simulink model "malt_mot_test"  (R2023a)
settings: Solver=FixedStepAuto  StartTime=0.0  StopTime=50  FixedStep=framePeriod_s  RelTol=1e-3
undefined symbols (not defined in the file or in its folder): Aircraft, framePeriod_s
settings Model: Creator=brian  LastModifiedBy=tuan
settings SolverCC: AlgebraicLoopSolver=TrustRegion
settings OptimizationCC: DefaultParameterBehavior=Inlined  GainParamInheritBuiltInType=on  UseFloatMulNetSlope=on  DefaultUnderspecifiedDataType=single  EnhancedBackFolding=on  BooleansAsBitfields=on  PassReuseOutputArgsAs=Individual arguments  StateBitsets=on  DataBitsets=on  ActiveStateOutputEnumStorageType=uint16  ZeroExternalMemoryAtStartup=off  ZeroInternalMemoryAtStartup=off  EfficientFloat2IntCast=on  LifeSpan=inf  DifferentSizesBufferReuse=on  OptimizationPriority=RAM  OptimizationCustomize=off  EfficientTunableParamExpr=on
settings DebuggingCC: ParameterPrecisionLossMsg=none  ParameterTunabilityLossMsg=error  UnconnectedInputMsg=warning  UnconnectedOutputMsg=warning  UnconnectedLineMsg=warning  BusObjectLabelMismatch=error  RootOutportRequireBusObject=error  NonBusSignalsTreatedAsBus=error  SFInvalidInputDataAccessInChartInitDiag=error  SFTransitionOutsideNaturalParentDiag=error  SFUnreachableExecutionPathDiag=error  SFUndirectedBroadcastEventsDiag=error
settings HardwareCC: ProdBitPerPointer=32  ProdBitPerSizeT=32  ProdBitPerPtrDiffT=32  ProdLargestAtomicInteger=Long  ProdLargestAtomicFloat=Double  ProdWordSize=32  ProdHWDeviceType=NXP->Cortex-M4  TargetLargestAtomicInteger=Long  TargetLargestAtomicFloat=Double  TargetLongLongMode=on  TargetIntDivRoundTo=Zero  TargetEndianess=LittleEndian  TargetHWDeviceType=NXP->Cortex-M4  ProdEqTarget=off
settings ModelReferenceCC: EnableRefExpFcnMdlSchedulingChecks=on  ModelReferenceNumInstancesAllowed=Single
settings SFSimCC: SimParseCustomCode=off  SimGenImportedTypeDefs=on  MATLABDynamicMemAlloc=off  SimTargetLang=C++
settings SFSimCC: SimUserIncludeDirs=|
  | ../../flight_code/include
  | ../../../ua_spaaro_extra/imu/include
  | ../../../ua_spaaro_extra/gnss/include
  | ../../../ua_spaaro_extra/pres/include
  | ../../../ua_spaaro_extra/sbus/include
  | ../../../ua_spaaro_extra/global_defs/include
settings SFSimCC: SimUserDefines=|
  | SIL
  | __FMU_R_MINI_V1__
settings RTWCC: Description=Embedded Coder  SystemTargetFile=ert.tlc  GenCodeOnly=on  TemplateMakefile=ert_default_tmf  GenerateReport=on  RTWVerbose=off  RTWUseSimCustomCode=on  Toolchain=GNU gcc/g++ | gmake (64-bit Linux)  BuildConfiguration=Specify  IncludeHyperlinkInReport=on  LaunchReport=on  TargetLang=C++  GenerateTraceInfo=on  GenerateTraceReport=on  GenerateTraceReportSl=on  GenerateTraceReportSf=on  GenerateTraceReportEml=on  GenerateCodeReplacementReport=on  DLArmComputeVersion=19.05
settings RTWCC: CustomInclude=|
  | ../../flight_code/include
  | ../../../ua_spaaro_extra/imu/include
  | ../../../ua_spaaro_extra/gnss/include
  | ../../../ua_spaaro_extra/pres/include
  | ../../../ua_spaaro_extra/sbus/include
  | ../../../ua_spaaro_extra/global_defs/include
settings RTWCC: CustomDefine=|
  | SIL
  | __FMU_R_MINI_V1__
settings CodeAppCC: ForceParamTrailComments=on  IgnoreCustomStorageClasses=off  OperatorAnnotations=on  SimulinkDataObjDesc=on  SFDataObjDesc=on  MATLABFcnDesc=on  CustomSymbolStrGlobalVar=rt$N$M  CustomSymbolStrType=$N$M  CustomSymbolStrFcn=$N$M$F  CustomSymbolStrMacro=$N$M  InsertBlockDesc=on  StateflowObjectComments=on  MATLABSourceComments=on  EnableCustomComments=on  InternalIdentifier=Classic  InlinedPrmAccess=Macros  ReqsInCode=on
settings ERTTargetCC: TargetLangStandard=C++03 (ISO)  GenerateFullHeader=off  IncludeMdlTerminateFcn=off  CombineSignalStateStructs=on  SuppressErrorStatus=on  SupportAbsoluteTime=off  CodeInterfacePackaging=C++ class  SupportNonFinite=off  SupportComplex=off  ParenthesesLevel=Standards  CastingMode=Standards  ERTHeaderFileRootName=autocode$E  ERTSourceFileRootName=autocode$E  InlinedParameterPlacement=NonHierarchical  RootIOFormat=Structure reference  ERTCustomFileTemplate=example_file_process.tlc  ERTFilePackagingFormat=Compact  PreserveExpressionOrder=on  PreserveIfCondition=on  ConvertIfToSwitch=off  EnableSignedLeftShifts=off  EnableSignedRightShifts=off  IndentSize=4

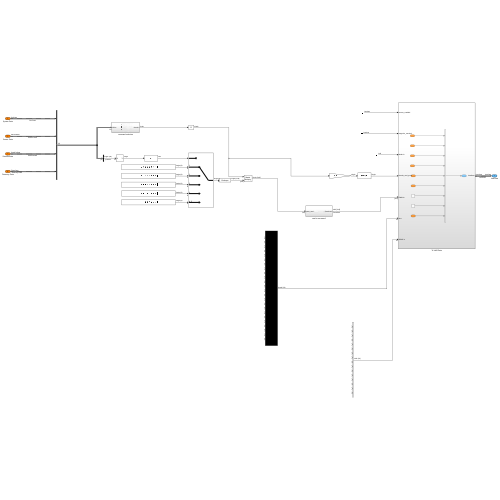
[thumbnail: Simulink's stored preview of the top-level diagram]
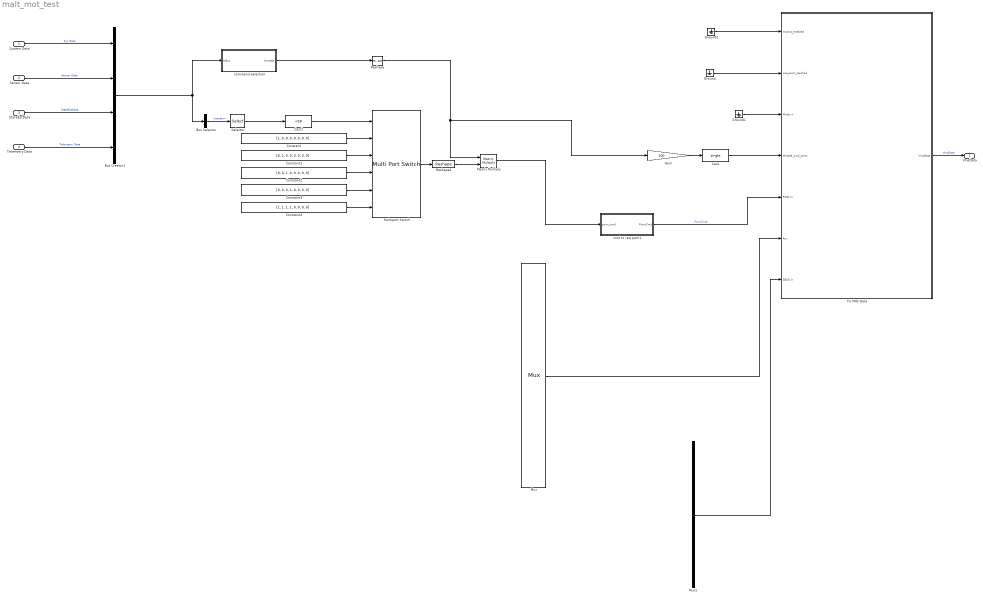
== system malt_mot_test ==
  System Data : Inport  OutDataTypeStr=Bus: SysData  SampleTime=framePeriod_s  BusOutputAsStruct=on
  Sensor Data : Inport  Port=2  OutDataTypeStr=Bus: SensorData  SampleTime=framePeriod_s  BusOutputAsStruct=on
  StateEstData : Inport  Port=3  OutDataTypeStr=Bus: StateEstData  SampleTime=framePeriod_s  BusOutputAsStruct=on
  Telemetry Data : Inport  Port=4  OutDataTypeStr=Bus: TelemData  SampleTime=framePeriod_s  BusOutputAsStruct=on
  Bus Creator1 : BusCreator  Inputs=4
  Bus Selector : BusSelector  OutputSignals=Telemetry Data.param
  Cast : DataTypeConversion  OutDataTypeStr=single  SaturateOnIntegerOverflow=off  RndMeth=Floor
  Cast1 : DataTypeConversion  OutDataTypeStr=int8  SaturateOnIntegerOverflow=off  RndMeth=Floor
  Constant : Constant  Value=[1, 0, 0, 0, 0, 0, 0, 0]  OutDataTypeStr=single  SampleTime=framePeriod_s
  Constant1 : Constant  Value=[0, 1, 0, 0, 0, 0, 0, 0]  OutDataTypeStr=single  SampleTime=framePeriod_s
  Constant2 : Constant  Value=[0, 0, 1, 0, 0, 0, 0, 0]  OutDataTypeStr=single  SampleTime=framePeriod_s
  Constant3 : Constant  Value=[0, 0, 0, 1, 0, 0, 0, 0]  OutDataTypeStr=single  SampleTime=framePeriod_s
  Constant4 : Constant  Value=[1, 1, 1, 1, 0, 0, 0, 0]  OutDataTypeStr=single  SampleTime=framePeriod_s
  Gain : Gain  Gain=100
  Ground : Ground
  Ground1 : Ground
  Ground2 : Ground
  Matrix Multiply : Product  Multiplication=Matrix(*)
  Multiport Switch : MultiPortSwitch  DataPortOrder=Specify indices  DataPortIndices={1, 2, 3, 4, 0}  SaturateOnIntegerOverflow=off  InputSameDT=off
  Mux : Mux  Inputs=24
  Mux1 : Mux  Inputs=16
  Reshape : Reshape  OutputDimensionality=Customize
  Reshape1 : Reshape  OutputDimensionality=Customize  OutputDimensions=[1,8]
  Selector : Selector  IndexMode=Zero-based  InputPortWidth=24  IndexOptions=Index vector (dialog)  Indices=0  OutputSizes=1
  To VMS Data : Subsystem
  cmd to raw pwm1 : Subsystem
  command selection : Subsystem
  VmsData : Outport  OutDataTypeStr=Bus: VmsData  SampleTime=framePeriod_s  BusOutputAsStruct=on
  wires:
  To VMS Data/1(VmsData) -> VmsData/1  "VmsData"
  Ground1/1 -> To VMS Data/3(Mode in)
  Ground2/1 -> To VMS Data/1(motors_enabled)
  Cast/1 -> To VMS Data/4(throttle_cmd_prcnt)
  Reshape/1 -> Gain/1, Matrix Multiply/1
  Gain/1 -> Cast/1
  command selection/1(throttle) -> Reshape/1
  Bus Creator1/1 -> Bus Selector/1, command selection/1(InBus)
  cmd to raw pwm1/1(PwmCmd) -> To VMS Data/5(PWM In)  "PwmCmd"
  Matrix Multiply/1 -> cmd to raw pwm1/1(pwm_cmd)
  Mux/1 -> To VMS Data/6(Aux)
  System Data/1 -> Bus Creator1/1  "Sys Data"
  Sensor Data/1 -> Bus Creator1/2  "Sensor Data"
  StateEstData/1 -> Bus Creator1/3  "StateEstData"
  Mux1/1 -> To VMS Data/7(SBUS in)
  Telemetry Data/1 -> Bus Creator1/4  "Telemetry Data"
  Ground/1 -> To VMS Data/2(waypoint_reached)
  Bus Selector/1 -> Selector/1  "<param>"
  Selector/1 -> Cast1/1
  Constant/1 -> Multiport Switch/2
  Constant1/1 -> Multiport Switch/3
  Constant4/1 -> Multiport Switch/6
  Constant3/1 -> Multiport Switch/5
  Constant2/1 -> Multiport Switch/4
  Multiport Switch/1 -> Reshape1/1
  Cast1/1 -> Multiport Switch/1
  Reshape1/1 -> Matrix Multiply/2

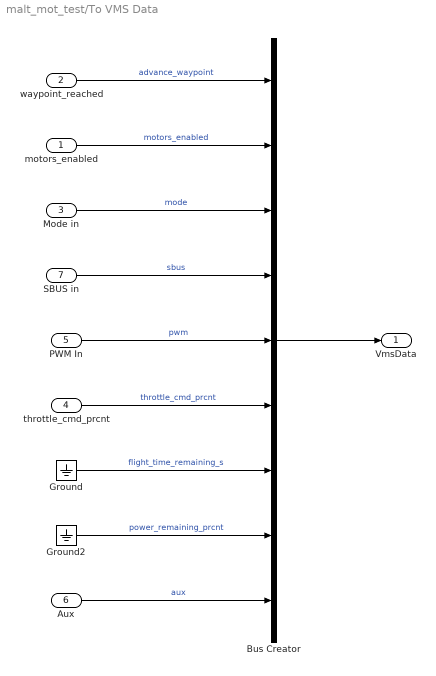
== system malt_mot_test/To VMS Data ==
  motors_enabled : Inport
  waypoint_reached : Inport  Port=2
  Mode in : Inport  Port=3
  throttle_cmd_prcnt : Inport  Port=4
  PWM In : Inport  Port=5
  Aux : Inport  Port=6
  SBUS in : Inport  Port=7
  Bus Creator : BusCreator  Inputs=9  OutDataTypeStr=Bus: VmsData  NonVirtualBus=on
      settings: InheritFromInputs=off
  Ground : Ground
  Ground2 : Ground
  VmsData : Outport
  wires:
  Bus Creator/1 -> VmsData/1
  waypoint_reached/1 -> Bus Creator/1  "advance_waypoint"
  motors_enabled/1 -> Bus Creator/2  "motors_enabled"
  Mode in/1 -> Bus Creator/3  "mode"
  SBUS in/1 -> Bus Creator/4  "sbus"
  PWM In/1 -> Bus Creator/5  "pwm"
  throttle_cmd_prcnt/1 -> Bus Creator/6  "throttle_cmd_prcnt"
  Aux/1 -> Bus Creator/9  "aux"
  Ground/1 -> Bus Creator/7  "flight_time_remaining_s"
  Ground2/1 -> Bus Creator/8  "power_remaining_prcnt"

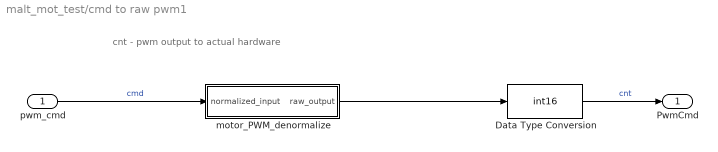
== system malt_mot_test/cmd to raw pwm1 ==
  note: cnt - pwm output to actual hardware
  pwm_cmd : Inport
  Data Type Conversion : DataTypeConversion  OutDataTypeStr=int16  SaturateOnIntegerOverflow=off  RndMeth=Floor
  motor_PWM_denormalize : Subsystem
  PwmCmd : Outport
  wires:
  pwm_cmd/1 -> motor_PWM_denormalize/1(normalized_input)  "cmd"
  motor_PWM_denormalize/1(raw_output) -> Data Type Conversion/1
  Data Type Conversion/1 -> PwmCmd/1  "cnt"

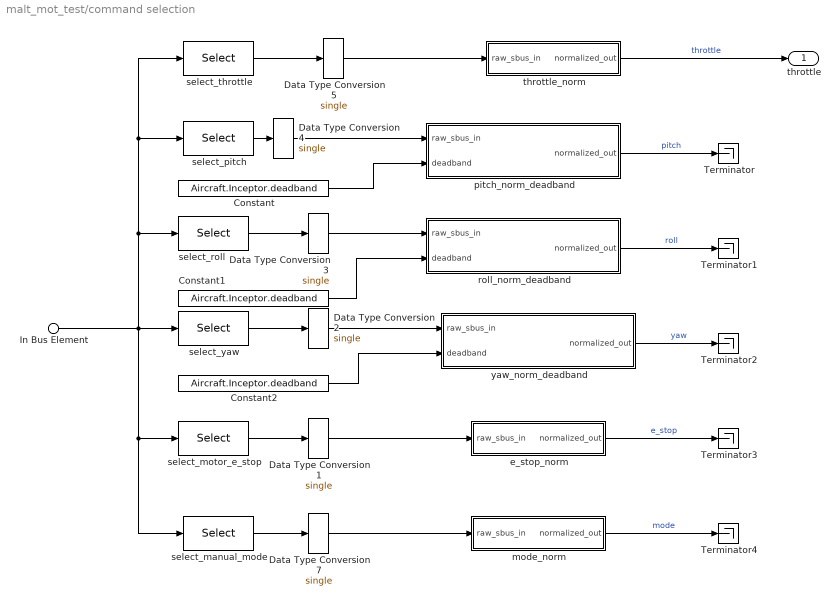
== system malt_mot_test/command selection ==
  In Bus Element : Inport  PortName=InBus  Element=Sensor Data.inceptor.ch
  Constant : Constant  Value=Aircraft.Inceptor.deadband  OutDataTypeStr=single
  Constant1 : Constant  Value=Aircraft.Inceptor.deadband  OutDataTypeStr=single
  Constant2 : Constant  Value=Aircraft.Inceptor.deadband  OutDataTypeStr=single
  Data Type Conversion{1..5,7} (6 alike) : DataTypeConversion  OutDataTypeStr=single  SaturateOnIntegerOverflow=off  RndMeth=Floor
  Terminator{,1..4} (5 alike) : Terminator
  e_stop_norm : Subsystem
  mode_norm : Subsystem
  pitch_norm_deadband : Subsystem
  roll_norm_deadband : Subsystem
  select_manual_mode : Selector  IndexOptions=Index vector (dialog)  Indices=Aircraft.Inceptor.mode0  OutputSizes=1
  select_motor_e_stop : Selector  IndexOptions=Index vector (dialog)  Indices=Aircraft.Inceptor.throttle_e_stop  OutputSizes=1
  select_pitch : Selector  IndexOptions=Index vector (dialog)  Indices=Aircraft.Inceptor.pitch  OutputSizes=1
  select_roll : Selector  IndexOptions=Index vector (dialog)  Indices=Aircraft.Inceptor.roll  OutputSizes=1
  select_throttle : Selector  IndexOptions=Index vector (dialog)  Indices=Aircraft.Inceptor.throttle  OutputSizes=1
  select_yaw : Selector  IndexOptions=Index vector (dialog)  Indices=Aircraft.Inceptor.yaw  OutputSizes=1
  throttle_norm : Subsystem
  yaw_norm_deadband : Subsystem
  throttle : Outport
  wires:
  select_pitch/1 -> Data Type Conversion4/1
  select_yaw/1 -> Data Type Conversion2/1
  select_throttle/1 -> Data Type Conversion5/1
  Data Type Conversion5/1 -> throttle_norm/1(raw_sbus_in)
  select_roll/1 -> Data Type Conversion3/1
  In Bus Element/1 -> select_roll/1, select_throttle/1, select_pitch/1, select_manual_mode/1, select_motor_e_stop/1, select_yaw/1
  Data Type Conversion1/1 -> e_stop_norm/1(raw_sbus_in)
  select_motor_e_stop/1 -> Data Type Conversion1/1
  Data Type Conversion7/1 -> mode_norm/1(raw_sbus_in)
  select_manual_mode/1 -> Data Type Conversion7/1
  Data Type Conversion2/1 -> yaw_norm_deadband/1(raw_sbus_in)
  Constant2/1 -> yaw_norm_deadband/2(deadband)
  throttle_norm/1(normalized_out) -> throttle/1  "throttle"
  roll_norm_deadband/1(normalized_out) -> Terminator1/1  "roll"
  pitch_norm_deadband/1(normalized_out) -> Terminator/1  "pitch"
  Data Type Conversion4/1 -> pitch_norm_deadband/1(raw_sbus_in)
  Constant/1 -> pitch_norm_deadband/2(deadband)
  Constant1/1 -> roll_norm_deadband/2(deadband)
  Data Type Conversion3/1 -> roll_norm_deadband/1(raw_sbus_in)
  yaw_norm_deadband/1(normalized_out) -> Terminator2/1  "yaw"
  e_stop_norm/1(normalized_out) -> Terminator3/1  "e_stop"
  mode_norm/1(normalized_out) -> Terminator4/1  "mode"

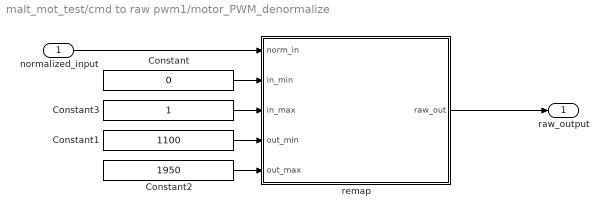
== system malt_mot_test/cmd to raw pwm1/motor_PWM_denormalize ==
  normalized_input : Inport
  Constant : Constant  Value=0  OutDataTypeStr=single
  Constant1 : Constant  Value=1100  OutDataTypeStr=single
  Constant2 : Constant  Value=1950  OutDataTypeStr=single
  Constant3 : Constant  OutDataTypeStr=single
  remap : MATLAB Function  TreatAsAtomicUnit=on
  raw_output : Outport
  wires:
  Constant2/1 -> remap/5(out_max)
  Constant1/1 -> remap/4(out_min)
  Constant3/1 -> remap/3(in_max)
  Constant/1 -> remap/2(in_min)
  remap/1(raw_out) -> raw_output/1
  normalized_input/1 -> remap/1(norm_in)

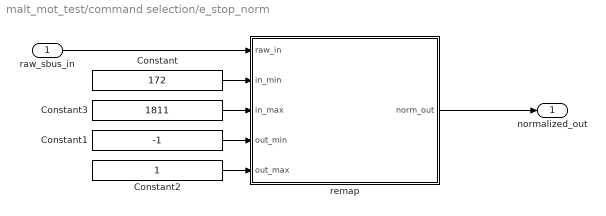
== system malt_mot_test/command selection/e_stop_norm ==
  raw_sbus_in : Inport
  Constant : Constant  Value=172  OutDataTypeStr=single
  Constant1 : Constant  Value=-1  OutDataTypeStr=single
  Constant2 : Constant  OutDataTypeStr=single
  Constant3 : Constant  Value=1811  OutDataTypeStr=single
  remap : MATLAB Function  TreatAsAtomicUnit=on
  normalized_out : Outport
  wires:
  Constant2/1 -> remap/5(out_max)
  Constant1/1 -> remap/4(out_min)
  Constant3/1 -> remap/3(in_max)
  Constant/1 -> remap/2(in_min)
  remap/1(norm_out) -> normalized_out/1
  raw_sbus_in/1 -> remap/1(raw_in)

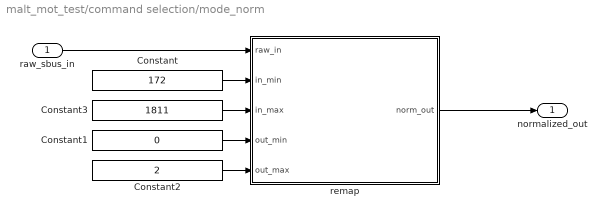
== system malt_mot_test/command selection/mode_norm ==
  raw_sbus_in : Inport
  Constant : Constant  Value=172  OutDataTypeStr=single
  Constant1 : Constant  Value=0  OutDataTypeStr=single
  Constant2 : Constant  Value=2  OutDataTypeStr=single
  Constant3 : Constant  Value=1811  OutDataTypeStr=single
  remap : MATLAB Function  TreatAsAtomicUnit=on
  normalized_out : Outport
  wires:
  raw_sbus_in/1 -> remap/1(raw_in)
  remap/1(norm_out) -> normalized_out/1
  Constant/1 -> remap/2(in_min)
  Constant3/1 -> remap/3(in_max)
  Constant1/1 -> remap/4(out_min)
  Constant2/1 -> remap/5(out_max)

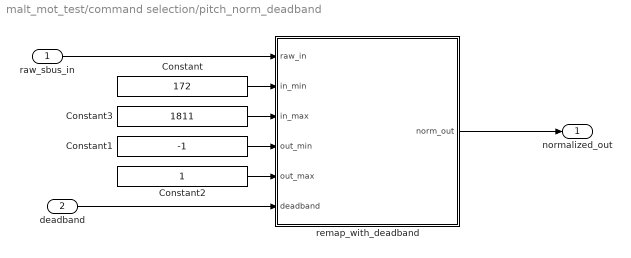
== system malt_mot_test/command selection/pitch_norm_deadband ==
  raw_sbus_in : Inport
  deadband : Inport  Port=2
  Constant : Constant  Value=172  OutDataTypeStr=single
  Constant1 : Constant  Value=-1  OutDataTypeStr=single
  Constant2 : Constant  OutDataTypeStr=single
  Constant3 : Constant  Value=1811  OutDataTypeStr=single
  remap_with_deadband : MATLAB Function  TreatAsAtomicUnit=on
  normalized_out : Outport
  wires:
  deadband/1 -> remap_with_deadband/6(deadband)
  Constant2/1 -> remap_with_deadband/5(out_max)
  Constant1/1 -> remap_with_deadband/4(out_min)
  Constant3/1 -> remap_with_deadband/3(in_max)
  Constant/1 -> remap_with_deadband/2(in_min)
  remap_with_deadband/1(norm_out) -> normalized_out/1
  raw_sbus_in/1 -> remap_with_deadband/1(raw_in)

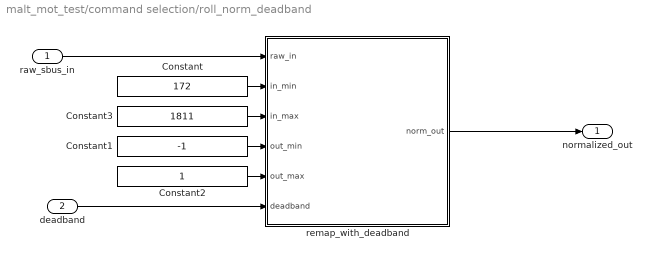
== system malt_mot_test/command selection/roll_norm_deadband ==
  raw_sbus_in : Inport
  deadband : Inport  Port=2
  Constant : Constant  Value=172  OutDataTypeStr=single
  Constant1 : Constant  Value=-1  OutDataTypeStr=single
  Constant2 : Constant  OutDataTypeStr=single
  Constant3 : Constant  Value=1811  OutDataTypeStr=single
  remap_with_deadband : MATLAB Function  TreatAsAtomicUnit=on
  normalized_out : Outport
  wires:
  deadband/1 -> remap_with_deadband/6(deadband)
  Constant2/1 -> remap_with_deadband/5(out_max)
  Constant1/1 -> remap_with_deadband/4(out_min)
  Constant3/1 -> remap_with_deadband/3(in_max)
  Constant/1 -> remap_with_deadband/2(in_min)
  remap_with_deadband/1(norm_out) -> normalized_out/1
  raw_sbus_in/1 -> remap_with_deadband/1(raw_in)

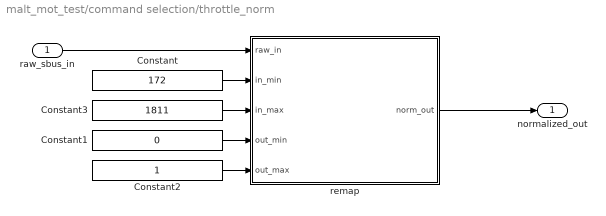
== system malt_mot_test/command selection/throttle_norm ==
  raw_sbus_in : Inport
  Constant : Constant  Value=172  OutDataTypeStr=single
  Constant1 : Constant  Value=0  OutDataTypeStr=single
  Constant2 : Constant  OutDataTypeStr=single
  Constant3 : Constant  Value=1811  OutDataTypeStr=single
  remap : MATLAB Function  TreatAsAtomicUnit=on
  normalized_out : Outport
  wires:
  raw_sbus_in/1 -> remap/1(raw_in)
  remap/1(norm_out) -> normalized_out/1
  Constant/1 -> remap/2(in_min)
  Constant3/1 -> remap/3(in_max)
  Constant1/1 -> remap/4(out_min)
  Constant2/1 -> remap/5(out_max)

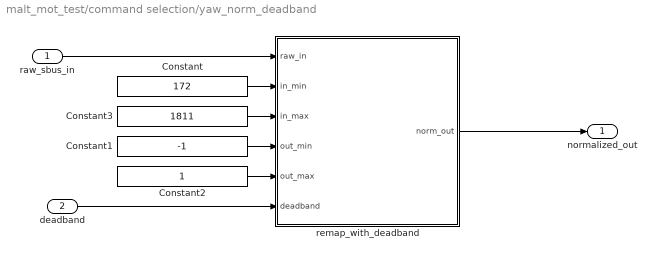
== system malt_mot_test/command selection/yaw_norm_deadband ==
  raw_sbus_in : Inport
  deadband : Inport  Port=2
  Constant : Constant  Value=172  OutDataTypeStr=single
  Constant1 : Constant  Value=-1  OutDataTypeStr=single
  Constant2 : Constant  OutDataTypeStr=single
  Constant3 : Constant  Value=1811  OutDataTypeStr=single
  remap_with_deadband : MATLAB Function  TreatAsAtomicUnit=on
  normalized_out : Outport
  wires:
  raw_sbus_in/1 -> remap_with_deadband/1(raw_in)
  remap_with_deadband/1(norm_out) -> normalized_out/1
  Constant/1 -> remap_with_deadband/2(in_min)
  Constant3/1 -> remap_with_deadband/3(in_max)
  Constant1/1 -> remap_with_deadband/4(out_min)
  Constant2/1 -> remap_with_deadband/5(out_max)
  deadband/1 -> remap_with_deadband/6(deadband)

== matlab function malt_mot_test/command selection/yaw_norm_deadband/remap_with_deadband ==
  data: raw_in input; norm_out output; in_min input; in_max input; out_min input; out_max input; deadband input
function norm_out = remap_deadband(raw_in, in_min, in_max, out_min, out_max, deadband)
in_avg = (in_min + in_max) / 2;
out_avg = (out_min + out_max) / 2;

in_deadband_range = (in_max - in_min) * deadband / 2;
in_deadband_low = in_avg - in_deadband_range;
in_deadband_hi = in_avg + in_deadband_range;

if raw_in < in_deadband_low
    norm_out = (raw_in - in_deadband_low) .* (out_max - out_avg)./(in_deadband_low - in_min) + out_avg;
elseif raw_in > in_deadband_low && raw_in < in_deadband_hi
    norm_out = out_avg;
else
    norm_out = (raw_in - in_deadband_hi) .* (out_max - out_avg)./(in_max - in_deadband_hi) + out_avg;
end

== matlab function malt_mot_test/command selection/throttle_norm/remap ==
  data: raw_in input; norm_out output; in_min input; in_max input; out_min input; out_max input
function norm_out = remap(raw_in,in_min,in_max,out_min,out_max)
norm_out = (raw_in - in_min) * (out_max - out_min)/(in_max-in_min) + out_min;

== matlab function malt_mot_test/command selection/roll_norm_deadband/remap_with_deadband ==
  data: raw_in input; norm_out output; in_min input; in_max input; out_min input; out_max input; deadband input
function norm_out = remap_deadband(raw_in, in_min, in_max, out_min, out_max, deadband)
in_avg = (in_min + in_max) / 2;
out_avg = (out_min + out_max) / 2;

in_deadband_range = (in_max - in_min) * deadband / 2;
in_deadband_low = in_avg - in_deadband_range;
in_deadband_hi = in_avg + in_deadband_range;

if raw_in < in_deadband_low
    norm_out = (raw_in - in_deadband_low) .* (out_max - out_avg)./(in_deadband_low - in_min) + out_avg;
elseif raw_in > in_deadband_low && raw_in < in_deadband_hi
    norm_out = out_avg;
else
    norm_out = (raw_in - in_deadband_hi) .* (out_max - out_avg)./(in_max - in_deadband_hi) + out_avg;
end

== matlab function malt_mot_test/command selection/pitch_norm_deadband/remap_with_deadband ==
  data: raw_in input; norm_out output; in_min input; in_max input; out_min input; out_max input; deadband input
function norm_out = remap_deadband(raw_in, in_min, in_max, out_min, out_max, deadband)
in_avg = (in_min + in_max) / 2;
out_avg = (out_min + out_max) / 2;

in_deadband_range = (in_max - in_min) * deadband / 2;
in_deadband_low = in_avg - in_deadband_range;
in_deadband_hi = in_avg + in_deadband_range;

if raw_in < in_deadband_low
    norm_out = (raw_in - in_deadband_low) .* (out_max - out_avg)./(in_deadband_low - in_min) + out_avg;
elseif raw_in > in_deadband_low && raw_in < in_deadband_hi
    norm_out = out_avg;
else
    norm_out = (raw_in - in_deadband_hi) .* (out_max - out_avg)./(in_max - in_deadband_hi) + out_avg;
end

== matlab function malt_mot_test/command selection/e_stop_norm/remap ==
  data: raw_in input; norm_out output; in_min input; in_max input; out_min input; out_max input
function norm_out = remap(raw_in,in_min,in_max,out_min,out_max)
norm_out = (raw_in - in_min) * (out_max - out_min)/(in_max-in_min) + out_min;

== matlab function malt_mot_test/command selection/mode_norm/remap ==
  data: raw_in input; norm_out output; in_min input; in_max input; out_min input; out_max input
function norm_out = remap(raw_in,in_min,in_max,out_min,out_max)
norm_out = (raw_in - in_min) * (out_max - out_min)/(in_max-in_min) + out_min;

== matlab function malt_mot_test/cmd to raw pwm1/motor_PWM_denormalize/remap ==
  data: norm_in input; raw_out output; in_min input; in_max input; out_min input; out_max input
function raw_out = remap(norm_in,in_min,in_max,out_min,out_max)
raw_out = (norm_in - in_min) * (out_max - out_min)/(in_max-in_min) + out_min;
